simulink model "chardonnay_simulinkR2019a"  (R2019a)
settings: Solver=VariableStepAuto  StartTime=0.0  StopTime=30  RelTol=1e-3
values from neighbouring files (symbols this model uses):
  K = (M*inv(V))    [level.m]    (also in main.m; poles_notes.m = [     -2.2361   -2.2361   -3.1109   -2.1804   19.2981    8.2)
settings Model: Creator=l.ribeiro-lustosa  LastModifiedBy=l.ribeiro-lustosa
settings DebuggingCC: SFMachineParentedDataDiag=error

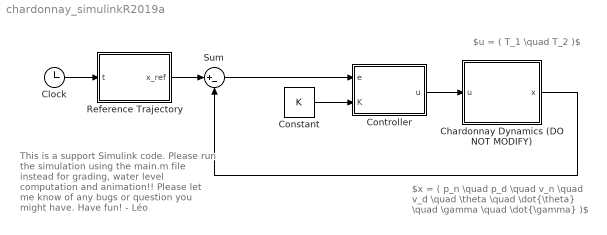
== system chardonnay_simulinkR2019a ==
  note: $x = ( p_n \quad p_d \quad v_n \quad v_d \quad \theta \quad \dot{\theta} \quad \gamma \quad \dot{\gamma} )$
  note: $u = ( T_1 \quad T_2 )$
  note: This is a support Simulink code.
      | Please run the simulation using the
      | main.m file instead for grading,
      | water level computation and animation!!
      |
      | Please let me know of any bugs or
      | question you might have.
      |
      | Have fun!
      | - Léo
  Chardonnay Dynamics (DO NOT MODIFY) : Subsystem
  Clock : Clock
  Constant : Constant  Value=K
  Controller : MATLAB Function  TreatAsAtomicUnit=on
  Reference Trajectory : MATLAB Function  TreatAsAtomicUnit=on
  Sum : Sum  Inputs=|+-
  wires:
  Chardonnay Dynamics (DO NOT MODIFY)/1(x) -> Sum/2
  Clock/1 -> Reference Trajectory/1(t)
  Reference Trajectory/1(x_ref) -> Sum/1
  Sum/1 -> Controller/1(e)
  Constant/1 -> Controller/2(K)
  Controller/1(u) -> Chardonnay Dynamics (DO NOT MODIFY)/1(u)

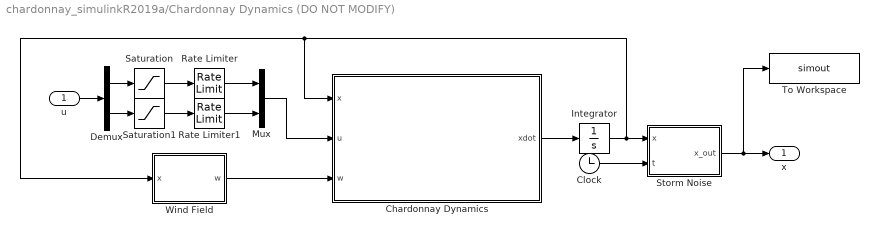
== system chardonnay_simulinkR2019a/Chardonnay Dynamics (DO NOT MODIFY) ==
  u : Inport
  Chardonnay Dynamics : MATLAB Function  TreatAsAtomicUnit=on
  Clock : Clock
  Demux : Demux  Outputs=2
  Integrator : Integrator  InitialCondition=zeros(8,1)
  Mux : Mux  Inputs=2
  Rate Limiter : RateLimiter  RisingSlewLimit=100  FallingSlewLimit=-100  SampleTimeMode=inherited
  Rate Limiter1 : RateLimiter  RisingSlewLimit=100  FallingSlewLimit=-100  SampleTimeMode=inherited
  Saturation : Saturate  UpperLimit=30  LowerLimit=0
  Saturation1 : Saturate  UpperLimit=30  LowerLimit=0
  Storm Noise : MATLAB Function  TreatAsAtomicUnit=on
  To Workspace : ToWorkspace  VariableName=simout  SaveFormat=Timeseries  SampleTime=1/30
  Wind Field : MATLAB Function  TreatAsAtomicUnit=on
  x : Outport
  wires:
  Chardonnay Dynamics/1(xdot) -> Integrator/1
  Integrator/1 -> Wind Field/1(x), Chardonnay Dynamics/1(x), Storm Noise/1(x)
  Wind Field/1(w) -> Chardonnay Dynamics/3(w)
  Storm Noise/1(x_out) -> To Workspace/1, x/1
  Clock/1 -> Storm Noise/2(t)
  u/1 -> Demux/1
  Saturation/1 -> Rate Limiter/1
  Saturation1/1 -> Rate Limiter1/1
  Demux/1 -> Saturation/1
  Demux/2 -> Saturation1/1
  Rate Limiter/1 -> Mux/1
  Rate Limiter1/1 -> Mux/2
  Mux/1 -> Chardonnay Dynamics/2(u)

== matlab function chardonnay_simulinkR2019a/Chardonnay Dynamics (DO NOT MODIFY)/Wind Field ==
  data: x input; w output
function w = wind_field(x)
% x = (pn, pd, vn, vd, the, thed, gam, gamd)

WIND_SPEED = 2;

pn = x(1);

if ( abs(pn-30)<5 )
    w = [0;WIND_SPEED];
else
    w = zeros(2,1);
end

== matlab function chardonnay_simulinkR2019a/Chardonnay Dynamics (DO NOT MODIFY)/Chardonnay Dynamics ==
  data: x input; u input; w input; xdot output
%% definition of equations of motion in nonlinear form
% this goes according to BE1, in the TA notes

function xdot = chardonnay_dynamics_s(x,u,w)
% x = (pn, pd, vn, vd, the, thed, gam, gamd)
% u = (T1, T2)
% w = (w1, w2)

chardonnay.m_d = 1;
chardonnay.m_c = 1;
chardonnay.l = 1;
chardonnay.l_d = 1;
chardonnay.J = 0.1;
chardonnay.C_D = 0.1;
chardonnay.g = 10;

m_d = chardonnay.m_d;
m_c = chardonnay.m_c;
l = chardonnay.l;
l_d = chardonnay.l_d;
J = chardonnay.J;
C_D = chardonnay.C_D;
g = chardonnay.g;

x_1 = x(3);
x_2 = x(4);
x_3 = x(5);
x_4 = x(6);
x_5 = x(7);
x_6 = x(8);

u_1 = u(1);
u_2 = u(2);

w_1 = w(1);
w_2 = w(2);

Pi = [
    m_d  0  0  0  0  0  sin(x_3+x_5);
    0  m_d  0  0  0  0  cos(x_3+x_5);
    m_c 0   0  -m_c*l*cos(x_3+x_5)  0  -m_c*l*cos(x_3+x_5)  -sin(x_3+x_5);
    0 m_c 0 m_c*l*sin(x_3+x_5) 0 m_c*l*sin(x_3+x_5)  -cos(x_3+x_5);
    0 0 0 J 0 0 0;
    0 0 1 0 0 0 0;
    0 0 0 0 1 0 0 ];

h = [
    -(u_1+u_2)*sin(x_3)-C_D*(x_1-w_1);
    m_d*g-(u_1+u_2)*cos(x_3)-C_D*(x_2-w_2);
    -m_c*l*(x_4+x_6)^2*sin(x_3+x_5);
    m_c*g-m_c*l*(x_4+x_6)^2*cos(x_3+x_5);
    (u_2-u_1)*l_d;
    x_4;
    x_6 ];

fp = Pi\h;
% drop the vinculum forces in the following!
f = fp(1:6);
% add position derivatives in the following!
xdot = [x_1;x_2;f];

end

== matlab function chardonnay_simulinkR2019a/Chardonnay Dynamics (DO NOT MODIFY)/Storm Noise ==
  data: x input; x_out output; t input
function x_out = storm(x,t)
% x = (pn, pd, vn, vd, the, thed, gam, gamd)

POS_NOISE = 0.1;
VEL_NOISE = 0.1;
ANG_NOISE = 3*pi/180;
ANG_VEL_NOISE = 0;

NOISE_FREQ_HZ = 1000;

pn = x(1);

if ( abs(pn-10)<5 )
    x_out = x + [POS_NOISE;POS_NOISE;VEL_NOISE;VEL_NOISE;ANG_NOISE;ANG_VEL_NOISE;ANG_NOISE;ANG_VEL_NOISE]*sin(2*pi*NOISE_FREQ_HZ*t);
else
    x_out = x;
end

== matlab function chardonnay_simulinkR2019a/Reference Trajectory ==
  data: t input; x_ref output
function x_ref = fcn(t)
% x = (pn, pd, vn, vd, the, thed, gam, gamd)

x_ref = zeros(8,1);

TIME_CTE = 10;

if (t<TIME_CTE)
    x_ref(1) = t/TIME_CTE*20;
    x_ref(2) = 10*sin( x_ref(1)/20*2*pi );
    x_ref(3) = 1/TIME_CTE*20;
    x_ref(4) = 10/20*2*pi*cos( x_ref(1)/20*2*pi );
elseif (t<2*TIME_CTE)
    x_ref(1) = 20+(t-TIME_CTE)/TIME_CTE*20;
    x_ref(3) = 1/TIME_CTE*20;
else
    x_ref(1) = 40;
    x_ref(3) = 0;
end

== matlab function chardonnay_simulinkR2019a/Controller ==
  data: e input; u output; K input
function u = fcn(e,K)
u = [10;10] + K*e;
